simulink model "DMA_throttle_sysgen_configurable_24a"  (R2024a)
settings: Solver=FixedStepAuto  StartTime=0.0  StopTime=300/125e6  FixedStep=1/125e6  RelTol=1e-3
model workspace (MAT data in the model file):
  Ts = 8e-09
undefined symbols (not defined in the file or in its folder): AXI4, Lite, xc7z020clg400
libraries: hdlBasic x59, simulink x10, vmcUtilities x1
settings Model: Creator=CDS-vmlynar
settings SolverCC: AlgebraicLoopSolver=TrustRegion
settings OptimizationCC: ReuseModelBlockBuffer=off
settings DebuggingCC: UnconnectedInputMsg=warning  UnconnectedOutputMsg=warning  UnconnectedLineMsg=warning
settings ModelReferenceCC: EnableRefExpFcnMdlSchedulingChecks=on
settings RTWCC: GPUComputeCapability=3.5  DLArmComputeVersion=19.05

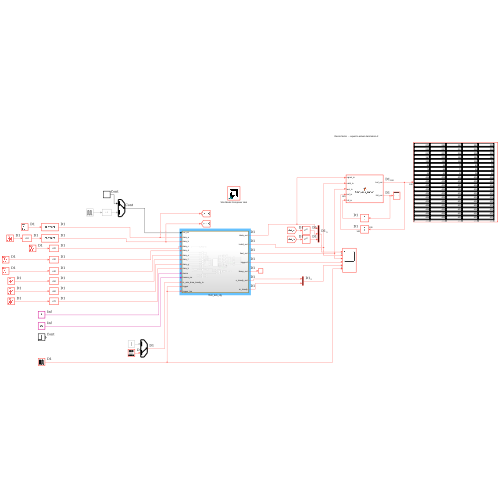
[thumbnail: Simulink's stored preview of the top-level diagram]
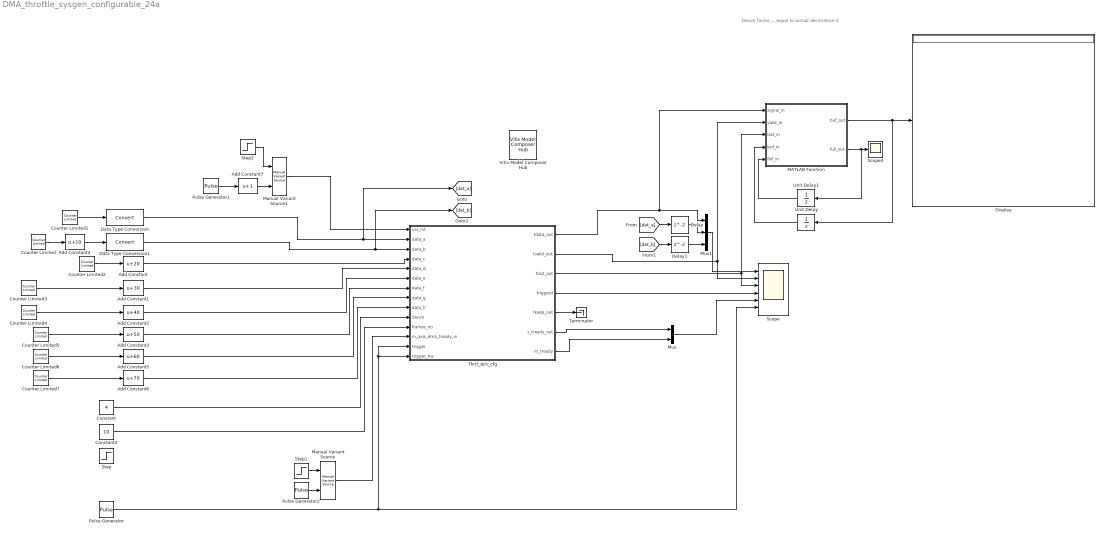
== system DMA_throttle_sysgen_configurable_24a ==
  note: Decim factor ... equal to actual decimation-2
  Add Constant : Bias  Bias=20  SaturateOnIntegerOverflow=off
  Add Constant1 : Bias  Bias=30  SaturateOnIntegerOverflow=off
  Add Constant2 : Bias  Bias=40  SaturateOnIntegerOverflow=off
  Add Constant3 : Bias  Bias=50  SaturateOnIntegerOverflow=off
  Add Constant4 : Bias  Bias=10  SaturateOnIntegerOverflow=off
  Add Constant5 : Bias  Bias=60  SaturateOnIntegerOverflow=off
  Add Constant6 : Bias  Bias=70  SaturateOnIntegerOverflow=off
  Add Constant7 : Bias  Bias=1  SaturateOnIntegerOverflow=off
  Constant : Constant  Value=4
  Constant2 : Constant  Value=10
  Counter Limited{,1..7} (8 alike) : simulink/Sources/Counter Limited  uplimit=4e9  tsamp=Ts
  Data Type Conversion : DataTypeConversion  SaturateOnIntegerOverflow=off  RndMeth=Floor
  Data Type Conversion1 : DataTypeConversion  SaturateOnIntegerOverflow=off  RndMeth=Floor
  Delay : Delay
  Delay1 : Delay
  Display : Display
  MATLAB Function : MATLAB Function  TreatAsAtomicUnit=on
  Manual Variant Source : simulink/Signal Routing/Manual Variant Source  NumChoices=2  LabelModeActiveChoice=V_2
  Manual Variant Source1 : simulink/Signal Routing/Manual Variant Source  NumChoices=2  LabelModeActiveChoice=V_1
  Mux : Mux  Inputs=2
  Mux1 : Mux  Inputs=3
  Pulse Generator : DiscretePulseGenerator  PulseType=Time based  Period=80/125e6  PulseWidth=5  PhaseDelay=10/125e6
  Pulse Generator1 : DiscretePulseGenerator  PulseType=Time based  Amplitude=-1  Period=80/125e6  PulseWidth=80  PhaseDelay=10/125e6
  Pulse Generator2 : DiscretePulseGenerator  Period=70  PulseWidth=44  PhaseDelay=40  SampleTime=Ts
  Scope : Scope  NumInputPorts=6
  Scope3 : Scope
  Step : Step  Time=10/125e6  SampleTime=0
  Step1 : Step  Time=20/125e6  SampleTime=Ts
  Step2 : Step  Time=5/125e6  Before=1  After=0  SampleTime=0
  Terminator : Terminator
  Thrtl_8ch_cfg : Subsystem
  Unit Delay : UnitDelay  InitialCondition=404*ones(100,1)  SampleTime=Ts  HasFrameUpgradeWarning=on
  Unit Delay1 : UnitDelay  SampleTime=Ts  HasFrameUpgradeWarning=on
  Vitis Model Composer Hub : vmcUtilities/Vitis Model Composer Hub  Tag=genX  CodeGeneration=off  SubsystemName=Thrtl_8ch_cfg  CompilationType=HDLCompilation  SubsystemType=HDLNode  ExportTypeV2=IP Catalog  StartColumn=1  NumberOfColumns=1  TargetDirectory=./netlist  exportDesign=on  analyzeDesign=off  validateDesignOnHw=off  ExportType=System Generator  IpVendor=xilinx.com  IpLibrary=hls  IpVersion=1.0  IpHWLanguage=Verilog  AieCompilerOptions={}  AieSimulatorOptions={}  CreateTestbench=off  TestbenchStackSize=10  RunRtlSim=off  RunCSim=off  RunAieSim=off  AieSimTimeout=50000  RunAieSimProfiling=off  LaunchVitisAnalyzer=off  PlotOutput=off  RunX86Sim=off  X86SimTimeout=10  GenHwImage=off  GenLibadfXo=off  GenHwValidationCode=off  PlatformType=Not Specified  HwSystemType=Baremetal  HwValidationTarget=hw  ProjDevice=xc7z020clg400-1  ProjDevicePart=xc7z020clg400-1  AIEType=None  SamplePeriod=-1  ClockFrequency=200  DataPathParallelism=1  xilinxfamily=zynq  part=xc7z020  speed=-1  package=clg400  directory=./netlist/ip/Thrtl_8ch_cfg/src  testbench=off  incr_netlist=off  synthesis_tool=Vivado  clock_wrapper=Clock Enables  dbl_ovrd=According to Block Masks  dcm_input_clock_period=10  sysclk_period=8  simulink_period=8e-9  eval_field=0  IPInfoJsonString="{\"DUTSubsystemName\":\"Thrtl_8ch_cfg\",\"HDLSubsystem\":{\"SubsystemName\":\"Thrtl_8ch_cfg\",\"IPName\":\"Thrtl_8ch_cfg\",\"IPLibrary\":\"VMC\",\"IPVendor\":\"User Company\",\"IPVersion\":\"1.0\",\"TargetDirectory\":\"./netlist\",\"SubsystemDir\":\"./netlist/ip/Thrtl_8ch_cfg\",\"FreqHz\":\"125000000\"},\"SubsystemTag\":\"HDLNode\"}"  LogFileName=/home/user/host_home/work/acin/projects/universal_lqg/lqg-fp7-firmware/dma_throttle/netlist/model_composer.log  NThreads=4  IPConfigFile=/tmp/vmctmp-user/10/ipconfig.json
  wires:
  Counter Limited1/1 -> Data Type Conversion/1
  Add Constant4/1 -> Data Type Conversion1/1
  Counter Limited2/1 -> Add Constant/1
  Counter Limited3/1 -> Add Constant1/1
  Counter Limited5/1 -> Add Constant3/1
  Counter Limited4/1 -> Add Constant2/1
  Counter Limited/1 -> Add Constant4/1
  Counter Limited6/1 -> Add Constant5/1
  Counter Limited7/1 -> Add Constant6/1
  Mux/1 -> Scope/5
  Add Constant7/1 -> Manual Variant Source1/2
  Pulse Generator1/1 -> Add Constant7/1
  Step1/1 -> Manual Variant Source/1
  Pulse Generator2/1 -> Manual Variant Source/2
  Pulse Generator/1 -> Thrtl_8ch_cfg/14(trigger_hw), Thrtl_8ch_cfg/13(trigger), Scope/6
  Step2/1 -> Manual Variant Source1/1
  Unit Delay1/1 -> MATLAB Function/5(full_in)
  MATLAB Function/2(full_out) -> Unit Delay1/1, Scope3/1
  Unit Delay/1 -> MATLAB Function/4(buf_in)
  MATLAB Function/1(buf_out) -> Display/1, Unit Delay/1
  Mux1/1 -> Scope/1
  Delay1/1 -> Mux1/3
  Delay/1 -> Mux1/2
  [dat_b] -> Delay1/1
  [dat_a] -> Delay/1
  Thrtl_8ch_cfg/2(tvalid_out) -> Scope/2, MATLAB Function/2(valid_in)
  Thrtl_8ch_cfg/1(tdata_out) -> MATLAB Function/1(signal_in), Mux1/1
  Thrtl_8ch_cfg/3(tlast_out) -> Scope/3, MATLAB Function/3(last_in)
  Manual Variant Source1/1 -> Thrtl_8ch_cfg/1(usr_rst)
  Add Constant/1 -> Thrtl_8ch_cfg/4(data_c)
  Add Constant1/1 -> Thrtl_8ch_cfg/5(data_d)
  Add Constant2/1 -> Thrtl_8ch_cfg/6(data_e)
  Add Constant3/1 -> Thrtl_8ch_cfg/7(data_f)
  Add Constant5/1 -> Thrtl_8ch_cfg/8(data_g)
  Add Constant6/1 -> Thrtl_8ch_cfg/9(data_h)
  Constant/1 -> Thrtl_8ch_cfg/10(decim)
  Constant2/1 -> Thrtl_8ch_cfg/11(frames_no)
  Manual Variant Source/1 -> Thrtl_8ch_cfg/12(m_axis_dma_tready_in)
  Thrtl_8ch_cfg/4(triggerd) -> Scope/4
  Thrtl_8ch_cfg/5(tkeep_out) -> Terminator/1
  Thrtl_8ch_cfg/6(s_tready_out) -> Mux/1
  Thrtl_8ch_cfg/7(m_tready) -> Mux/2
  Data Type Conversion/1 -> [dat_a], Thrtl_8ch_cfg/2(data_a)
  Data Type Conversion1/1 -> [dat_b], Thrtl_8ch_cfg/3(data_b)

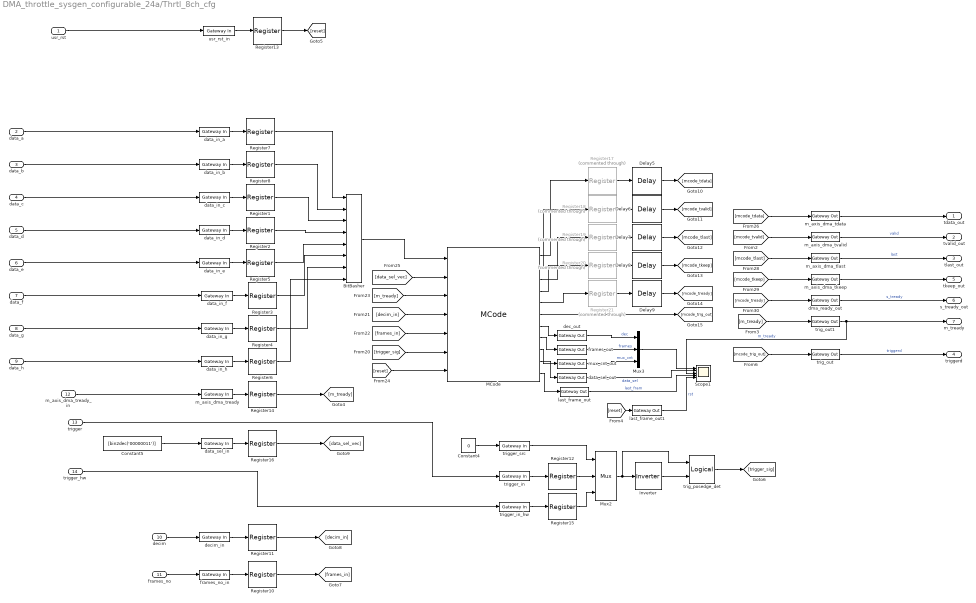
== system DMA_throttle_sysgen_configurable_24a/Thrtl_8ch_cfg ==
  usr_rst : Inport
  data_a : Inport  Port=2
  data_b : Inport  Port=3
  data_c : Inport  Port=4
  data_d : Inport  Port=5
  data_e : Inport  Port=6
  data_f : Inport  Port=7
  data_g : Inport  Port=8
  data_h : Inport  Port=9
  decim : Inport  Port=10
  frames_no : Inport  Port=11
  m_axis_dma_tready_in : Inport  Port=12
  trigger : Inport  Port=13
  trigger_hw : Inport  Port=14
  BitBasher : hdlBasic/BitBasher  bitexpr=out={h,g,f,e,d,c,b,a}  display_expr=off  sr_1=out  arith_type1=Unsigned  bin_pt1=0  sr_2=2  arith_type2=Unsigned  bin_pt2=0  sr_3=3  arith_type3=Unsigned  bin_pt3=0  sr_4=4  arith_type4=Unsigned  bin_pt4=0  XmcBlockStatus=1  maskContainerNames=group1  block_type=bitbasher  block_config=sysgen:BitBasher_config
  Constant4 : Constant  Value=0
  Constant5 : Constant  Value=[bin2dec('00000011')]
  Delay{5..9} (5 alike) : hdlBasic/Delay  rst=off  en=off  latency=1  reg_retiming=on  XmcBlockStatus=1  maskContainerNames=group1  block_type=delay  block_config=sysgen:Delay_config
  Inverter : hdlBasic/Inverter  en=off  latency=1  XmcBlockStatus=1  maskContainerNames=group2  block_type=inv  block_config=sysgen:Inverter_config
  MCode : hdlBasic/MCode  mfname=throttle_core  explicit_period=on  period=Ts  iptable={'data_vec','';'data_sel','';'tready_in','';'decim_val','';'frames_val','';'trigger_in','';'usr_rst','';'AXIS_WIDTH','32';'NO_CHANNELS','8'}  optable={'tdata','off';'tvalid','off';'tlast','off';'tkeep','off';'tready','off';'trigger_out','off';'dec_cnt_out','off';'frame_cnt_out','off';'mux_cnt_out','off';'data_sel_out','off';'last_frame_out','off'}  enable_stdout=off  enable_debug=off  suppress_output=on  defparams={'AXIS_WIDTH',32,'NO_CHANNELS',8}  hide_port_list={}  block_type=mcode  block_width=444  block_height=788
      settings: infoedit=Pass input values to a MATLAB function for evaluation in Xilinx fixed-point type. The input ports of the block are input arguments of the function. The output ports of the block are output arguments of the function.
  Mux2 : hdlBasic/Mux  inputs=2  en=off  latency=1  precision=Full  arith_type=Unsigned  n_bits=16  bin_pt=14  quantization=Truncate  overflow=Wrap  XmcBlockStatus=1  maskContainerNames=tabcontainer1  block_type=mux  block_config=sysgen:Mux_config
  Mux3 : Mux  Inputs=3
  Register{1..8,10..16} (15 alike) : hdlBasic/Register  init=0  rst=off  en=off  XmcBlockStatus=1  maskContainerNames=tabcontainer1  block_type=register  block_config=sysgen:Register_config
  Register{17..21} (5 alike) : hdlBasic/Register  Commented=through  init=0  rst=off  en=off  XmcBlockStatus=1  maskContainerNames=tabcontainer1  block_type=register  block_config=sysgen:Register_config
  Scope1 : Scope  NumInputPorts=5
  data_in_a : hdlBasic/Gateway In  gui_display_data_type=Fixed-point  arith_type=Unsigned  n_bits=32  bin_pt=0  preci_type=Single  exp_width=8  frac_width=24  rows=1  columns=1  quantization="Round  (unbiased: +/- Inf)"  overflow=Saturate  period=1/125e6  UseAsADC=off  ADCChannel='1'  interface=None  automatic_assignment=on  address_offset=hex2dec('00')  intf_name=''  intf_description=''  default_value=0  timing_constraint=None  locs_specified=off  LOCs={}  io_standard={}  inherit_from_input=off  hdl_port=on  XmcBlockStatus=1  maskContainerNames=group4  block_type=gatewayin  block_config=sysgen:gateway_in_config  block_width_w=590  block_height_w=620  block_width=640  block_height=850
  data_in_b : hdlBasic/Gateway In  gui_display_data_type=Fixed-point  arith_type=Unsigned  n_bits=32  bin_pt=0  preci_type=Single  exp_width=8  frac_width=24  rows=1  columns=1  quantization="Round  (unbiased: +/- Inf)"  overflow=Saturate  period=Ts  UseAsADC=off  ADCChannel='1'  interface=None  automatic_assignment=on  address_offset=hex2dec('00')  intf_name=''  intf_description=''  default_value=0  timing_constraint=None  locs_specified=off  LOCs={}  io_standard={}  inherit_from_input=off  hdl_port=on  XmcBlockStatus=1  maskContainerNames=group4  block_type=gatewayin  block_config=sysgen:gateway_in_config  block_width_w=590  block_height_w=620  block_width=640  block_height=850
  data_in_c : hdlBasic/Gateway In  gui_display_data_type=Fixed-point  arith_type=Unsigned  n_bits=32  bin_pt=0  preci_type=Single  exp_width=8  frac_width=24  rows=1  columns=1  quantization="Round  (unbiased: +/- Inf)"  overflow=Saturate  period=Ts  UseAsADC=off  ADCChannel='1'  interface=None  automatic_assignment=on  address_offset=hex2dec('00')  intf_name=''  intf_description=''  default_value=0  timing_constraint=None  locs_specified=off  LOCs={}  io_standard={}  inherit_from_input=off  hdl_port=on  XmcBlockStatus=1  maskContainerNames=group4  block_type=gatewayin  block_config=sysgen:gateway_in_config  block_width_w=590  block_height_w=620  block_width=640  block_height=850
  data_in_d : hdlBasic/Gateway In  gui_display_data_type=Fixed-point  arith_type=Unsigned  n_bits=32  bin_pt=0  preci_type=Single  exp_width=8  frac_width=24  rows=1  columns=1  quantization="Round  (unbiased: +/- Inf)"  overflow=Saturate  period=Ts  UseAsADC=off  ADCChannel='1'  interface=None  automatic_assignment=on  address_offset=hex2dec('00')  intf_name=''  intf_description=''  default_value=0  timing_constraint=None  locs_specified=off  LOCs={}  io_standard={}  inherit_from_input=off  hdl_port=on  XmcBlockStatus=1  maskContainerNames=group4  block_type=gatewayin  block_config=sysgen:gateway_in_config  block_width_w=590  block_height_w=620  block_width=640  block_height=850
  data_in_e : hdlBasic/Gateway In  gui_display_data_type=Fixed-point  arith_type=Unsigned  n_bits=32  bin_pt=0  preci_type=Single  exp_width=8  frac_width=24  rows=1  columns=1  quantization="Round  (unbiased: +/- Inf)"  overflow=Saturate  period=Ts  UseAsADC=off  ADCChannel='1'  interface=None  automatic_assignment=on  address_offset=hex2dec('00')  intf_name=''  intf_description=''  default_value=0  timing_constraint=None  locs_specified=off  LOCs={}  io_standard={}  inherit_from_input=off  hdl_port=on  XmcBlockStatus=1  maskContainerNames=group4  block_type=gatewayin  block_config=sysgen:gateway_in_config  block_width_w=590  block_height_w=620  block_width=640  block_height=850
  data_in_f : hdlBasic/Gateway In  gui_display_data_type=Fixed-point  arith_type=Unsigned  n_bits=32  bin_pt=0  preci_type=Single  exp_width=8  frac_width=24  rows=1  columns=1  quantization="Round  (unbiased: +/- Inf)"  overflow=Saturate  period=Ts  UseAsADC=off  ADCChannel='1'  interface=None  automatic_assignment=on  address_offset=hex2dec('00')  intf_name=''  intf_description=''  default_value=0  timing_constraint=None  locs_specified=off  LOCs={}  io_standard={}  inherit_from_input=off  hdl_port=on  XmcBlockStatus=1  maskContainerNames=group4  block_type=gatewayin  block_config=sysgen:gateway_in_config  block_width_w=590  block_height_w=620  block_width=640  block_height=850
  data_in_g : hdlBasic/Gateway In  gui_display_data_type=Fixed-point  arith_type=Unsigned  n_bits=32  bin_pt=0  preci_type=Single  exp_width=8  frac_width=24  rows=1  columns=1  quantization="Round  (unbiased: +/- Inf)"  overflow=Saturate  period=Ts  UseAsADC=off  ADCChannel='1'  interface=None  automatic_assignment=on  address_offset=hex2dec('00')  intf_name=''  intf_description=''  default_value=0  timing_constraint=None  locs_specified=off  LOCs={}  io_standard={}  inherit_from_input=off  hdl_port=on  XmcBlockStatus=1  maskContainerNames=group4  block_type=gatewayin  block_config=sysgen:gateway_in_config  block_width_w=590  block_height_w=620  block_width=640  block_height=850
  data_in_h : hdlBasic/Gateway In  gui_display_data_type=Fixed-point  arith_type=Unsigned  n_bits=32  bin_pt=0  preci_type=Single  exp_width=8  frac_width=24  rows=1  columns=1  quantization="Round  (unbiased: +/- Inf)"  overflow=Saturate  period=Ts  UseAsADC=off  ADCChannel='1'  interface=None  automatic_assignment=on  address_offset=hex2dec('00')  intf_name=''  intf_description=''  default_value=0  timing_constraint=None  locs_specified=off  LOCs={}  io_standard={}  inherit_from_input=off  hdl_port=on  XmcBlockStatus=1  maskContainerNames=group4  block_type=gatewayin  block_config=sysgen:gateway_in_config  block_width_w=590  block_height_w=620  block_width=640  block_height=850
  data_sel_in : hdlBasic/Gateway In  gui_display_data_type=Fixed-point  arith_type=Unsigned  n_bits=8  bin_pt=0  preci_type=Single  exp_width=8  frac_width=24  rows=1  columns=1  quantization="Round  (unbiased: +/- Inf)"  overflow=Wrap  period=Ts  UseAsADC=off  ADCChannel='1'  interface=AXI4-Lite  automatic_assignment=off  address_offset=hex2dec('14')  intf_name='cfg_in'  intf_description=''  default_value=3  timing_constraint=None  locs_specified=off  LOCs={}  io_standard={}  inherit_from_input=off  hdl_port=on  XmcBlockStatus=1  maskContainerNames=group4  block_type=gatewayin  block_config=sysgen:gateway_in_config  block_width_w=590  block_height_w=620  block_width=640  block_height=850
  data_sel_out : hdlBasic/Gateway Out  inherit_from_input=on  hdl_port=off  rows=1  columns=1  UseAsDAC=off  DACChannel='1'  interface=None  automatic_assignment=on  address_offset=hex2dec('00')  intf_name=''  intf_description=''  timing_constraint=None  locs_specified=off  LOCs={}  io_standard={}  XmcBlockStatus=1  maskContainerNames=group4  block_type=gatewayout  block_config=sysgen:gateway_out_config  block_width_w=590  block_height_w=620  block_width=620  block_height=750
  dec_out : hdlBasic/Gateway Out  inherit_from_input=off  hdl_port=off  rows=1  columns=1  UseAsDAC=off  DACChannel='1'  interface=None  automatic_assignment=on  address_offset=hex2dec('00')  intf_name=''  intf_description=''  timing_constraint=None  locs_specified=off  LOCs={}  io_standard={}  XmcBlockStatus=1  maskContainerNames=group4  block_type=gatewayout  block_config=sysgen:gateway_out_config  block_width_w=590  block_height_w=620  block_width=620  block_height=750
  decim_in : hdlBasic/Gateway In  gui_display_data_type=Fixed-point  arith_type=Unsigned  n_bits=16  bin_pt=0  preci_type=Single  exp_width=8  frac_width=24  rows=1  columns=1  quantization="Round  (unbiased: +/- Inf)"  overflow=Saturate  period=Ts  UseAsADC=off  ADCChannel='1'  interface=AXI4-Lite  automatic_assignment=off  address_offset=hex2dec('0C')  intf_name='cfg_in'  intf_description=''  default_value=0  timing_constraint=None  locs_specified=off  LOCs={}  io_standard={}  inherit_from_input=off  hdl_port=on  XmcBlockStatus=1  maskContainerNames=group4  block_type=gatewayin  block_config=sysgen:gateway_in_config  block_width_w=590  block_height_w=620  block_width=640  block_height=850
  dma_ready_out : hdlBasic/Gateway Out  inherit_from_input=on  hdl_port=on  rows=1  columns=1  UseAsDAC=off  DACChannel='1'  interface=None  automatic_assignment=on  address_offset=hex2dec('00')  intf_name=''  intf_description=''  timing_constraint=None  locs_specified=off  LOCs={}  io_standard={}  XmcBlockStatus=1  maskContainerNames=group4  block_type=gatewayout  block_config=sysgen:gateway_out_config  block_width_w=590  block_height_w=620  block_width=620  block_height=750
  frames_no_in : hdlBasic/Gateway In  gui_display_data_type=Fixed-point  arith_type=Unsigned  n_bits=32  bin_pt=0  preci_type=Single  exp_width=8  frac_width=24  rows=1  columns=1  quantization="Round  (unbiased: +/- Inf)"  overflow=Saturate  period=Ts  UseAsADC=off  ADCChannel='1'  interface=AXI4-Lite  automatic_assignment=off  address_offset=hex2dec('08')  intf_name='cfg_in'  intf_description=''  default_value=0  timing_constraint=None  locs_specified=off  LOCs={}  io_standard={}  inherit_from_input=off  hdl_port=on  XmcBlockStatus=1  maskContainerNames=group4  block_type=gatewayin  block_config=sysgen:gateway_in_config  block_width_w=590  block_height_w=620  block_width=640  block_height=850
  frames_out : hdlBasic/Gateway Out  inherit_from_input=off  hdl_port=off  rows=1  columns=1  UseAsDAC=off  DACChannel='1'  interface=None  automatic_assignment=on  address_offset=hex2dec('00')  intf_name=''  intf_description=''  timing_constraint=None  locs_specified=off  LOCs={}  io_standard={}  XmcBlockStatus=1  maskContainerNames=group4  block_type=gatewayout  block_config=sysgen:gateway_out_config  block_width_w=590  block_height_w=620  block_width=620  block_height=750
  last_frame_out : hdlBasic/Gateway Out  inherit_from_input=on  hdl_port=off  rows=1  columns=1  UseAsDAC=off  DACChannel='1'  interface=None  automatic_assignment=on  address_offset=hex2dec('00')  intf_name=''  intf_description=''  timing_constraint=None  locs_specified=off  LOCs={}  io_standard={}  XmcBlockStatus=1  maskContainerNames=group4  block_type=gatewayout  block_config=sysgen:gateway_out_config  block_width_w=590  block_height_w=620  block_width=620  block_height=750
  last_frame_out1 : hdlBasic/Gateway Out  inherit_from_input=on  hdl_port=off  rows=1  columns=1  UseAsDAC=off  DACChannel='1'  interface=None  automatic_assignment=on  address_offset=hex2dec('00')  intf_name=''  intf_description=''  timing_constraint=None  locs_specified=off  LOCs={}  io_standard={}  XmcBlockStatus=1  maskContainerNames=group4  block_type=gatewayout  block_config=sysgen:gateway_out_config  block_width_w=590  block_height_w=620  block_width=620  block_height=750
  m_axis_dma_tdata : hdlBasic/Gateway Out  inherit_from_input=off  hdl_port=on  rows=1  columns=1  UseAsDAC=off  DACChannel='1'  interface=None  automatic_assignment=on  address_offset=hex2dec('00')  intf_name=''  intf_description=''  timing_constraint=None  locs_specified=off  LOCs={}  io_standard={}  XmcBlockStatus=1  maskContainerNames=group4  block_type=gatewayout  block_config=sysgen:gateway_out_config  block_width_w=590  block_height_w=620  block_width=620  block_height=750
  m_axis_dma_tkeep : hdlBasic/Gateway Out  inherit_from_input=off  hdl_port=on  rows=1  columns=1  UseAsDAC=off  DACChannel='1'  interface=None  automatic_assignment=on  address_offset=hex2dec('00')  intf_name=''  intf_description=''  timing_constraint=None  locs_specified=off  LOCs={}  io_standard={}  XmcBlockStatus=1  maskContainerNames=group4  block_type=gatewayout  block_config=sysgen:gateway_out_config  block_width_w=590  block_height_w=620  block_width=620  block_height=750
  m_axis_dma_tlast : hdlBasic/Gateway Out  inherit_from_input=on  hdl_port=on  rows=1  columns=1  UseAsDAC=off  DACChannel='1'  interface=None  automatic_assignment=on  address_offset=hex2dec('00')  intf_name=''  intf_description=''  timing_constraint=None  locs_specified=off  LOCs={}  io_standard={}  XmcBlockStatus=1  maskContainerNames=group4  block_type=gatewayout  block_config=sysgen:gateway_out_config  block_width_w=590  block_height_w=620  block_width=620  block_height=750
  m_axis_dma_tready : hdlBasic/Gateway In  gui_display_data_type=Boolean  arith_type=Boolean  n_bits=1  bin_pt=0  preci_type=Single  exp_width=8  frac_width=24  rows=1  columns=1  quantization="Round  (unbiased: +/- Inf)"  overflow=Saturate  period=Ts  UseAsADC=off  ADCChannel='1'  interface=None  automatic_assignment=off  address_offset=hex2dec('00')  intf_name='cfg_in'  intf_description=''  default_value=0  timing_constraint=None  locs_specified=off  LOCs={}  io_standard={}  inherit_from_input=off  hdl_port=on  XmcBlockStatus=1  maskContainerNames=group4  block_type=gatewayin  block_config=sysgen:gateway_in_config  block_width_w=590  block_height_w=620  block_width=640  block_height=850
  m_axis_dma_tvalid : hdlBasic/Gateway Out  inherit_from_input=on  hdl_port=on  rows=1  columns=1  UseAsDAC=off  DACChannel='1'  interface=None  automatic_assignment=on  address_offset=hex2dec('00')  intf_name=''  intf_description=''  timing_constraint=None  locs_specified=off  LOCs={}  io_standard={}  XmcBlockStatus=1  maskContainerNames=group4  block_type=gatewayout  block_config=sysgen:gateway_out_config  block_width_w=590  block_height_w=620  block_width=620  block_height=750
  mux_cnt_out : hdlBasic/Gateway Out  inherit_from_input=off  hdl_port=off  rows=1  columns=1  UseAsDAC=off  DACChannel='1'  interface=None  automatic_assignment=on  address_offset=hex2dec('00')  intf_name=''  intf_description=''  timing_constraint=None  locs_specified=off  LOCs={}  io_standard={}  XmcBlockStatus=1  maskContainerNames=group4  block_type=gatewayout  block_config=sysgen:gateway_out_config  block_width_w=590  block_height_w=620  block_width=620  block_height=750
  trig_out : hdlBasic/Gateway Out  inherit_from_input=on  hdl_port=off  rows=1  columns=1  UseAsDAC=off  DACChannel='1'  interface=None  automatic_assignment=on  address_offset=hex2dec('00')  intf_name=''  intf_description=''  timing_constraint=None  locs_specified=off  LOCs={}  io_standard={}  XmcBlockStatus=1  maskContainerNames=group4  block_type=gatewayout  block_config=sysgen:gateway_out_config  block_width_w=590  block_height_w=620  block_width=620  block_height=750
  trig_out1 : hdlBasic/Gateway Out  inherit_from_input=on  hdl_port=off  rows=1  columns=1  UseAsDAC=off  DACChannel='1'  interface=None  automatic_assignment=on  address_offset=hex2dec('00')  intf_name=''  intf_description=''  timing_constraint=None  locs_specified=off  LOCs={}  io_standard={}  XmcBlockStatus=1  maskContainerNames=group4  block_type=gatewayout  block_config=sysgen:gateway_out_config  block_width_w=590  block_height_w=620  block_width=620  block_height=750
  trig_posedge_det : hdlBasic/Logical  logical_function=AND  inputs=2  en=off  latency=0  precision=Full  arith_type=Unsigned  n_bits=16  bin_pt=0  align_bp=on  overflow=[]  quantization=[]  XmcBlockStatus=1  maskContainerNames=tabcontainer1  block_type=logical  block_config=sysgen:Logical_config
  trigger_in : hdlBasic/Gateway In  gui_display_data_type=Boolean  arith_type=Boolean  n_bits=1  bin_pt=0  preci_type=Single  exp_width=8  frac_width=24  rows=1  columns=1  quantization="Round  (unbiased: +/- Inf)"  overflow=Saturate  period=Ts  UseAsADC=off  ADCChannel='1'  interface=AXI4-Lite  automatic_assignment=off  address_offset=hex2dec('00')  intf_name='cfg_in'  intf_description=''  default_value=0  timing_constraint=None  locs_specified=off  LOCs={}  io_standard={}  inherit_from_input=off  hdl_port=on  XmcBlockStatus=1  maskContainerNames=group4  block_type=gatewayin  block_config=sysgen:gateway_in_config  block_width_w=590  block_height_w=620  block_width=640  block_height=850
  trigger_in_hw : hdlBasic/Gateway In  gui_display_data_type=Boolean  arith_type=Boolean  n_bits=1  bin_pt=0  preci_type=Single  exp_width=8  frac_width=24  rows=1  columns=1  quantization="Round  (unbiased: +/- Inf)"  overflow=Saturate  period=Ts  UseAsADC=off  ADCChannel='1'  interface=None  automatic_assignment=off  address_offset=hex2dec('00')  intf_name='cfg_in'  intf_description=''  default_value=0  timing_constraint=None  locs_specified=off  LOCs={}  io_standard={}  inherit_from_input=off  hdl_port=on  XmcBlockStatus=1  maskContainerNames=group4  block_type=gatewayin  block_config=sysgen:gateway_in_config  block_width_w=590  block_height_w=620  block_width=640  block_height=850
  trigger_src : hdlBasic/Gateway In  gui_display_data_type=Boolean  arith_type=Boolean  n_bits=1  bin_pt=0  preci_type=Single  exp_width=8  frac_width=24  rows=1  columns=1  quantization="Round  (unbiased: +/- Inf)"  overflow=Saturate  period=Ts  UseAsADC=off  ADCChannel='1'  interface=AXI4-Lite  automatic_assignment=off  address_offset=hex2dec('10')  intf_name='cfg_in'  intf_description=''  default_value=0  timing_constraint=None  locs_specified=off  LOCs={}  io_standard={}  inherit_from_input=off  hdl_port=on  XmcBlockStatus=1  maskContainerNames=group4  block_type=gatewayin  block_config=sysgen:gateway_in_config  block_width_w=590  block_height_w=620  block_width=640  block_height=850
  usr_rst_in : hdlBasic/Gateway In  gui_display_data_type=Boolean  arith_type=Boolean  n_bits=1  bin_pt=0  preci_type=Single  exp_width=8  frac_width=24  rows=1  columns=1  quantization="Round  (unbiased: +/- Inf)"  overflow=Saturate  period=Ts  UseAsADC=off  ADCChannel='1'  interface=AXI4-Lite  automatic_assignment=off  address_offset=hex2dec('04')  intf_name='cfg_in'  intf_description=''  default_value=0  timing_constraint=None  locs_specified=off  LOCs={}  io_standard={}  inherit_from_input=off  hdl_port=on  XmcBlockStatus=1  maskContainerNames=group4  block_type=gatewayin  block_config=sysgen:gateway_in_config  block_width_w=590  block_height_w=620  block_width=640  block_height=850
  tdata_out : Outport
  tvalid_out : Outport  Port=2
  tlast_out : Outport  Port=3
  triggerd : Outport  Port=4
  tkeep_out : Outport  Port=5
  s_tready_out : Outport  Port=6
  m_tready : Outport  Port=7
  wires:
  Register15/1 -> Mux2/3
  Mux2/1 -> Inverter/1, trig_posedge_det/1
  MCode/4 -> Register20/1
  data_in_d/1 -> Register2/1
  Register10/1 -> [frames_in]
  frames_out/1 -> Mux3/2  "frames"
  frames_no_in/1 -> Register10/1
  data_c/1 -> data_in_c/1
  Register2/1 -> BitBasher/4
  usr_rst_in/1 -> Register13/1
  Inverter/1 -> trig_posedge_det/2
  [reset] -> last_frame_out1/1
  trigger_in/1 -> Register12/1
  [m_tready] -> trig_out1/1
  [mcode_tlast] -> m_axis_dma_tlast/1
  MCode/5 -> Register21/1
  Register7/1 -> BitBasher/1
  data_in_e/1 -> Register5/1
  trig_out1/1 -> Scope1/3, m_tready/1  "m_tready"
  Delay9/1 -> [mcode_tready]
  MCode/3 -> Register19/1
  Register13/1 -> [reset]
  [mcode_tvalid] -> m_axis_dma_tvalid/1
  data_e/1 -> data_in_e/1
  MCode/1 -> Register17/1
  data_sel_out/1 -> Scope1/2  "data_sel"
  Register14/1 -> [m_tready]
  MCode/11 -> last_frame_out/1
  last_frame_out/1 -> Scope1/4  "last_fram"
  Constant5/1 -> data_sel_in/1
  [mcode_tkeep] -> m_axis_dma_tkeep/1
  Register20/1 -> Delay8/1
  Register11/1 -> [decim_in]
  Register6/1 -> BitBasher/8
  MCode/8 -> frames_out/1
  Register19/1 -> Delay7/1
  Register16/1 -> [data_sel_vec]
  [trigger_sig] -> MCode/6
  [mcode_tready] -> dma_ready_out/1
  Delay6/1 -> [mcode_tvalid]
  trigger_src/1 -> Mux2/1
  Register17/1 -> Delay5/1
  Constant4/1 -> trigger_src/1
  trig_posedge_det/1 -> [trigger_sig]
  [mcode_tdata] -> m_axis_dma_tdata/1
  [decim_in] -> MCode/4
  Delay7/1 -> [mcode_tlast]
  Register3/1 -> BitBasher/6
  [data_sel_vec] -> MCode/2
  Register18/1 -> Delay6/1
  MCode/2 -> Register18/1
  Register8/1 -> BitBasher/2
  MCode/6 -> [mcode_trig_out]
  BitBasher/1 -> MCode/1
  m_axis_dma_tready/1 -> Register14/1
  [m_tready] -> MCode/3
  mux_cnt_out/1 -> Mux3/3  "mux_cnt"
  data_f/1 -> data_in_f/1
  data_sel_in/1 -> Register16/1
  Register1/1 -> BitBasher/3
  [reset] -> MCode/7
  Register5/1 -> BitBasher/5
  last_frame_out1/1 -> Scope1/5  "rst"
  Register12/1 -> Mux2/2
  [frames_in] -> MCode/5
  Register4/1 -> BitBasher/7
  Register21/1 -> Delay9/1
  Delay5/1 -> [mcode_tdata]
  Delay8/1 -> [mcode_tkeep]
  Mux3/1 -> Scope1/1
  MCode/9 -> mux_cnt_out/1
  MCode/10 -> data_sel_out/1
  dec_out/1 -> Mux3/1  "dec"
  MCode/7 -> dec_out/1
  data_in_h/1 -> Register6/1
  [mcode_trig_out] -> trig_out/1
  data_g/1 -> data_in_g/1
  trigger_in_hw/1 -> Register15/1
  decim_in/1 -> Register11/1
  data_in_a/1 -> Register7/1
  data_in_f/1 -> Register3/1
  data_in_c/1 -> Register1/1
  data_in_g/1 -> Register4/1
  data_a/1 -> data_in_a/1
  data_in_b/1 -> Register8/1
  data_b/1 -> data_in_b/1
  trigger/1 -> trigger_in/1
  m_axis_dma_tready_in/1 -> m_axis_dma_tready/1
  trigger_hw/1 -> trigger_in_hw/1
  m_axis_dma_tdata/1 -> tdata_out/1
  usr_rst/1 -> usr_rst_in/1
  dma_ready_out/1 -> s_tready_out/1  "s_tready"
  m_axis_dma_tlast/1 -> tlast_out/1  "last"
  m_axis_dma_tkeep/1 -> tkeep_out/1
  m_axis_dma_tvalid/1 -> tvalid_out/1  "valid"
  trig_out/1 -> triggerd/1  "triggerd"
  data_d/1 -> data_in_d/1
  decim/1 -> decim_in/1
  frames_no/1 -> frames_no_in/1
  data_h/1 -> data_in_h/1

== matlab function DMA_throttle_sysgen_configurable_24a/MATLAB Function ==
  data: signal_in input; buf_out output; valid_in input; last_in input; buf_in input; full_out output; full_in input
function [buf_out, full_out] = Sampling_buffer(signal_in, valid_in, last_in, buf_in, full_in)

if (valid_in == true) && (full_in == false)
    buf_in = circshift(buf_in,1);
    buf_in(1) = signal_in;
end

if (last_in == true)
    full_out = 1;
else
    full_out = full_in;
end

if (full_in == 1)
    full_out = 0;
end

buf_out = buf_in;
